simulink model "FinSimLagrange1"  (R2020b)
settings: Solver=FixedStepAuto  StartTime=0.0  StopTime=10.0  FixedStep=0.001  RelTol=1e-3
values from neighbouring files (symbols this model uses):
  m = {0 0 0 0 0}    [DynMatrixCalculator.m]    (also in DynMats_Iterative.mat = ; FinLagrange_2.m = mass{i})
  N = {zeros(3,1) zeros(3,1) zeros(3,1) zeros(3,1) zeros(3,1)}    [DynMatrixCalculator.m]    (also in DynMats_Iterative.mat = )
undefined symbols (not defined in the file or in its folder): X, Y, Z
libraries: sm_lib x34, nesl_utility x24
(part 3 of 4)

== matlab function FinSimLagrange1/Tau Iterative/MATLAB Function1 ==
  data: d2dt input; th2 input; th2dt input; th2ddt input; Force1 output; th3 input; th3dt input; th3ddt input; tau2 output; th4 input; th4dt input; th4ddt input; tau3 output; tau4 output
function [Force1, tau2, tau3, tau4] = fcn(d2dt, th2, th2dt, th2ddt, th3, th3dt, th3ddt, th4, th4dt, th4ddt)
% m0=cte(1); m1=cte(2); m2=cte(3); m3=cte(4); m4=cte(5); g=cte(6);
m0=40.117; m1=22.064; m2=9.805; m3=13.302; m4=10.723;
g=9.81;

%[Ixx Iyy Izz;Iyz Ixz Ixy]
Ic1=[13.366 13.428 .066;0 0 0];
Ic2=[.134 .165 .186;0 .001 -.012];
Ic3=[.082 .053 .058;-.001 0 0];
Ic4=[.048 .175 .153;0 .001 .003];
Ic5=[.018 .166 .164;0 -.001 .009];

Ixx0=Ic1(1,1);Ixx1=Ic2(1,1);Ixx2=Ic3(1,1);Ixx3=Ic4(1,1);Ixx4=Ic5(1,1);
Iyy0=Ic1(1,2);Iyy1=Ic2(1,2);Iyy2=Ic3(1,2);Iyy3=Ic4(1,2);Iyy4=Ic5(1,2);
Izz0=Ic1(1,3);Izz1=Ic2(1,3);Izz2=Ic3(1,3);Izz3=Ic4(1,3);Izz4=Ic5(1,3);
Iyz0=Ic1(2,1);Iyz1=Ic2(2,1);Iyz2=Ic3(2,1);Iyz3=Ic4(2,1);Iyz4=Ic5(2,1);
Ixz0=Ic1(2,2);Ixz1=Ic2(2,2);Ixz2=Ic3(2,2);Ixz3=Ic4(2,2);Ixz4=Ic5(2,2);
Ixy0=Ic1(2,3);Ixy1=Ic2(2,3);Ixy2=Ic3(2,3);Ixy3=Ic4(2,3);Ixy4=Ic5(2,3);

M=[0,                                                                                                                                                                                                                                                                                                                                                                                                                                                                                                                                                                      sin(th2)*(m3/1000 - m2/1000 + m4/1000) + cos(th2)*(m2/200 - (29*m3)/100 - (29*m4)/100 - (143*m4*cos(th3 + th4))/1000 + (3*m4*sin(th3 + th4))/200 + (11*m3*cos(th3))/1000 + (m4*cos(th3))/50 + (59*m3*sin(th3))/500 + (1913*m4*sin(th3))/5000),                                                                                                                                           (sin(th2)*(75*m4*cos(th3 + th4) + 715*m4*sin(th3 + th4) + 590*m3*cos(th3) + 1913*m4*cos(th3) - 55*m3*sin(th3) - 100*m4*sin(th3)))/5000,                                                                                                      (20674^(1/2)*m4*sin(th3 + th4 + atan(15/143))*sin(th2))/1000
0, Ixx3/2 + Ixx4/2 + Iyy3/2 + Iyy4/2 + Izz2 + (13*m2)/500000 + (17131*m3)/2500000 + (656439*m4)/10000000 - (13803*m3*cos(2*th3))/2000000 - (55477*m4*cos(2*th3))/1000000 - (Ixx4*cos(2*th3 + 2*th4))/2 + (Iyy4*cos(2*th3 + 2*th4))/2 + (649*m3*sin(2*th3))/500000 + (29*m4*sin(2*th3))/10000 + Ixy4*sin(2*th3 + 2*th4) + (158*m4*cos(2*th3 + 2*th4))/15625 - (429*m4*sin(2*th3 + 2*th4))/200000 + (4138563*m4*cos(th3 + th4))/100000000 - (86823*m4*sin(th3 + th4))/20000000 - (318351*m3*cos(th3))/100000000 + (59*m4*cos(th3))/5000000 + (7229*m4*cos(th4))/2000000 - (1707519*m3*sin(th3))/50000000 - (41937133*m4*sin(th3))/500000000 + (482409*m4*sin(th4))/10000000 - (12949*m4*cos(2*th3 + th4))/2000000 + (Ixx3*cos(2*th3))/2 - (Iyy3*cos(2*th3))/2 - (479409*m4*sin(2*th3 + th4))/10000000 - Ixy3*sin(2*th3), cos(th3)*(Ixz3 + (59*m3)/500000 + (1913*m4)/5000000 + Iyz4*cos(th4) + Ixz4*sin(th4) + (3*m4*cos(th4))/200000 + (143*m4*sin(th4))/1000000) - (sin(th3)*(1000000*Iyz3 + 11*m3 + 20*m4 - 1000000*Ixz4*cos(th4) + 1000000*Iyz4*sin(th4) - 143*m4*cos(th4) + 15*m4*sin(th4)))/1000000, sin(th3)*(cos(th4)*(Ixz4 + (143*m4)/1000000) - sin(th4)*(Iyz4 + (3*m4)/200000)) + cos(th3)*(cos(th4)*(Iyz4 + (3*m4)/200000) + sin(th4)*(Ixz4 + (143*m4)/1000000))
0,                                                                                                                                                                                                                                                                                                                                                                                                                                                                                                                                                                                          Iyz4*cos(th3 + th4) + Ixz4*sin(th3 + th4) + (3*m4*cos(th3 + th4))/200000 + Ixz3*cos(th3) + (143*m4*sin(th3 + th4))/1000000 - Iyz3*sin(th3) + (59*m3*cos(th3))/500000 + (29*m4*cos(th3))/100000 - (11*m3*sin(th3))/1000000,                                                                                                                                                                   Izz3 + Izz4 + (2809*m3)/200000 + (32907*m4)/250000 + (7229*m4*cos(th4))/1000000 + (482409*m4*sin(th4))/5000000,                                                                                     Izz4 + (10337*m4)/500000 + (87*m4*cos(th4))/20000 + (4147*m4*sin(th4))/100000
0,                                                                                                                                                                                                                                                                                                                                                                                                                                                                                                                                                                                                                                                                                                         Iyz4*cos(th3 + th4) + Ixz4*sin(th3 + th4) + (3*m4*cos(th3 + th4))/200000 + (143*m4*sin(th3 + th4))/1000000,                                                                                                                                                                                             Izz4 + (10337*m4)/500000 + (2879*m4*cos(th4))/1000000 + (275059*m4*sin(th4))/5000000,                                                                                                                                          Izz4 + (10337*m4)/500000];

V=[                                                                                                                                                                                                                                                                                  (m3*th2dt^2*cos(th2))/1000 - (m2*th2dt^2*cos(th2))/1000 + (m4*th2dt^2*cos(th2))/1000 - (m2*th2dt^2*sin(th2))/200 + (29*m3*th2dt^2*sin(th2))/100 + (29*m4*th2dt^2*sin(th2))/100 - (11*m3*th2dt^2*cos(th3)*sin(th2))/1000 - (11*m3*th3dt^2*cos(th3)*sin(th2))/1000 - (m4*th2dt^2*cos(th3)*sin(th2))/50 - (m4*th3dt^2*cos(th3)*sin(th2))/50 - (59*m3*th2dt^2*sin(th2)*sin(th3))/500 - (59*m3*th3dt^2*sin(th2)*sin(th3))/500 - (1913*m4*th2dt^2*sin(th2)*sin(th3))/5000 - (1913*m4*th3dt^2*sin(th2)*sin(th3))/5000 + (143*m4*th2dt^2*cos(th3)*cos(th4)*sin(th2))/1000 + (143*m4*th3dt^2*cos(th3)*cos(th4)*sin(th2))/1000 + (143*m4*th4dt^2*cos(th3)*cos(th4)*sin(th2))/1000 - (3*m4*th2dt^2*cos(th3)*sin(th2)*sin(th4))/200 - (3*m4*th2dt^2*cos(th4)*sin(th2)*sin(th3))/200 - (3*m4*th3dt^2*cos(th3)*sin(th2)*sin(th4))/200 - (3*m4*th3dt^2*cos(th4)*sin(th2)*sin(th3))/200 - (3*m4*th4dt^2*cos(th3)*sin(th2)*sin(th4))/200 - (3*m4*th4dt^2*cos(th4)*sin(th2)*sin(th3))/200 - (143*m4*th2dt^2*sin(th2)*sin(th3)*sin(th4))/1000 - (143*m4*th3dt^2*sin(th2)*sin(th3)*sin(th4))/1000 - (143*m4*th4dt^2*sin(th2)*sin(th3)*sin(th4))/1000 + (59*m3*th2dt*th3dt*cos(th2)*cos(th3))/250 + (1913*m4*th2dt*th3dt*cos(th2)*cos(th3))/2500 - (11*m3*th2dt*th3dt*cos(th2)*sin(th3))/500 - (m4*th2dt*th3dt*cos(th2)*sin(th3))/25 + (3*m4*th2dt*th3dt*cos(th2)*cos(th3)*cos(th4))/100 + (3*m4*th2dt*th4dt*cos(th2)*cos(th3)*cos(th4))/100 + (143*m4*th2dt*th3dt*cos(th2)*cos(th3)*sin(th4))/500 + (143*m4*th2dt*th3dt*cos(th2)*cos(th4)*sin(th3))/500 + (143*m4*th2dt*th4dt*cos(th2)*cos(th3)*sin(th4))/500 + (143*m4*th2dt*th4dt*cos(th2)*cos(th4)*sin(th3))/500 + (143*m4*th3dt*th4dt*cos(th3)*cos(th4)*sin(th2))/500 - (3*m4*th2dt*th3dt*cos(th2)*sin(th3)*sin(th4))/100 - (3*m4*th2dt*th4dt*cos(th2)*sin(th3)*sin(th4))/100 - (3*m4*th3dt*th4dt*cos(th3)*sin(th2)*sin(th4))/100 - (3*m4*th3dt*th4dt*cos(th4)*sin(th2)*sin(th3))/100 - (143*m4*th3dt*th4dt*sin(th2)*sin(th3)*sin(th4))/500
(29059*m3*th2dt^2)/100000000 + (29059*m4*th2dt^2)/100000000 + Ixz4*th3dt^2*cos(th3 + th4) + Ixz4*th4dt^2*cos(th3 + th4) - Iyz4*th3dt^2*sin(th3 + th4) - Iyz4*th4dt^2*sin(th3 + th4) + (143*m4*th3dt^2*cos(th3 + th4))/1000000 + (143*m4*th4dt^2*cos(th3 + th4))/1000000 - Iyz3*th3dt^2*cos(th3) - (3*m4*th3dt^2*sin(th3 + th4))/200000 - (3*m4*th4dt^2*sin(th3 + th4))/200000 - Ixz3*th3dt^2*sin(th3) - (11*m3*th3dt^2*cos(th3))/1000000 - (m4*th2dt^2*cos(th3))/50000 - (m4*th3dt^2*cos(th3))/50000 - (59*m3*th3dt^2*sin(th3))/500000 - (463*m4*th2dt^2*sin(th3))/5000000 - (1913*m4*th3dt^2*sin(th3))/5000000 - (29*m4*th2dt*th3dt)/5000 + Ixx4*th2dt*th3dt*sin(2*th3 + 2*th4) + Ixx4*th2dt*th4dt*sin(2*th3 + 2*th4) - Iyy4*th2dt*th3dt*sin(2*th3 + 2*th4) - Iyy4*th2dt*th4dt*sin(2*th3 + 2*th4) - (429*m4*th2dt*th3dt*cos(2*th3 + 2*th4))/100000 - (429*m4*th2dt*th4dt*cos(2*th3 + 2*th4))/100000 - (316*m4*th2dt*th3dt*sin(2*th3 + 2*th4))/15625 - (316*m4*th2dt*th4dt*sin(2*th3 + 2*th4))/15625 + 2*Ixz4*th3dt*th4dt*cos(th3 + th4) - 2*Iyz4*th3dt*th4dt*sin(th3 + th4) + (177*m4*th2dt*th3dt*cos(th3 + th4))/10000000 + (177*m4*th2dt*th4dt*cos(th3 + th4))/10000000 + (143*m4*th3dt*th4dt*cos(th3 + th4))/500000 + (8437*m4*th2dt*th3dt*sin(th3 + th4))/50000000 + (8437*m4*th2dt*th4dt*sin(th3 + th4))/50000000 - (3*m4*th3dt*th4dt*sin(th3 + th4))/100000 + (3481*m3*th2dt*th3dt*cos(th3))/25000000 + (112867*m4*th2dt*th3dt*cos(th3))/250000000 - (67709*m4*th2dt*th3dt*cos(th4))/5000000 + (4147*m4*th2dt*th4dt*cos(th4))/100000 - (649*m3*th2dt*th3dt*sin(th3))/50000000 - (59*m4*th2dt*th3dt*sin(th3))/2500000 - (1471*m4*th2dt*th3dt*sin(th4))/1000000 - (87*m4*th2dt*th4dt*sin(th4))/20000 - (479409*m4*th2dt*th3dt*cos(2*th3 + th4))/5000000 - (4147*m4*th2dt*th4dt*cos(2*th3 + th4))/100000 - 2*Ixy3*th2dt*th3dt*cos(2*th3) + (12949*m4*th2dt*th3dt*sin(2*th3 + th4))/1000000 + (87*m4*th2dt*th4dt*sin(2*th3 + th4))/20000 - Ixx3*th2dt*th3dt*sin(2*th3) + Iyy3*th2dt*th3dt*sin(2*th3) + (649*m3*th2dt*th3dt*cos(2*th3))/250000 + (29*m4*th2dt*th3dt*cos(2*th3))/5000 + 2*Ixy4*th2dt*th3dt*cos(2*th3 + 2*th4) + 2*Ixy4*th2dt*th4dt*cos(2*th3 + 2*th4) + (13803*m3*th2dt*th3dt*sin(2*th3))/1000000 + (55477*m4*th2dt*th3dt*sin(2*th3))/500000
                                                                                                                                                                                                                                                                                                                                                                                                                                                                                                                                                                                                                                                                                                                                                                                                                                                                                                                                                                                                                                                                                                                                                             (429*m4*th2dt^2*cos(2*th3 + 2*th4))/200000 - (29*m4*th3dt^2)/5000 - (29*m4*th2dt^2)/10000 + (158*m4*th2dt^2*sin(2*th3 + 2*th4))/15625 + (87*m4*th2dt^2*cos(th3 + th4))/20000 + (4147*m4*th2dt^2*sin(th3 + th4))/100000 + (1711*m3*th2dt^2*cos(th3))/50000 + (841*m4*th2dt^2*cos(th3))/10000 - (67709*m4*th2dt^2*cos(th4))/10000000 - (67709*m4*th3dt^2*cos(th4))/5000000 + (4147*m4*th4dt^2*cos(th4))/100000 - (319*m3*th2dt^2*sin(th3))/100000 - (1471*m4*th2dt^2*sin(th4))/2000000 - (1471*m4*th3dt^2*sin(th4))/1000000 - (87*m4*th4dt^2*sin(th4))/20000 + (479409*m4*th2dt^2*cos(2*th3 + th4))/10000000 + Ixy3*th2dt^2*cos(2*th3) - (12949*m4*th2dt^2*sin(2*th3 + th4))/2000000 + (Ixx3*th2dt^2*sin(2*th3))/2 - (Iyy3*th2dt^2*sin(2*th3))/2 - (649*m3*th2dt^2*cos(2*th3))/500000 - (29*m4*th2dt^2*cos(2*th3))/10000 - Ixy4*th2dt^2*cos(2*th3 + 2*th4) - (13803*m3*th2dt^2*sin(2*th3))/2000000 - (55477*m4*th2dt^2*sin(2*th3))/1000000 - (Ixx4*th2dt^2*sin(2*th3 + 2*th4))/2 + (Iyy4*th2dt^2*sin(2*th3 + 2*th4))/2 + (4147*m4*th3dt*th4dt*cos(th4))/50000 - (87*m4*th3dt*th4dt*sin(th4))/10000
                                                                                                                                                                                                                                                                                                                                                                                                                                                                                                                                                                                                                                                                                                                                                                                                                                                                                                                                                                                                                                                                                                                                                                                                                                                                                                                                                                                                                                                                                                                                                                                                                                                                                                                  (429*m4*th2dt^2*cos(2*th3 + 2*th4))/200000 + (158*m4*th2dt^2*sin(2*th3 + 2*th4))/15625 + (87*m4*th2dt^2*cos(th3 + th4))/20000 + (4147*m4*th2dt^2*sin(th3 + th4))/100000 - (275059*m4*th2dt^2*cos(th4))/10000000 - (275059*m4*th3dt^2*cos(th4))/5000000 + (2879*m4*th2dt^2*sin(th4))/2000000 + (2879*m4*th3dt^2*sin(th4))/1000000 + (272059*m4*th2dt^2*cos(2*th3 + th4))/10000000 - (8599*m4*th2dt^2*sin(2*th3 + th4))/2000000 - Ixy4*th2dt^2*cos(2*th3 + 2*th4) - (Ixx4*th2dt^2*sin(2*th3 + 2*th4))/2 + (Iyy4*th2dt^2*sin(2*th3 + 2*th4))/2];

G=[                                                                                                            0
                                                                                                            0
-(g*(15*m4*sin(th3 + th4) - 143*m4*cos(th3 + th4) + 11*m3*cos(th3) + 118*m3*sin(th3) + 290*m4*sin(th3)))/1000
                                                         (g*m4*(143*cos(th3 + th4) - 15*sin(th3 + th4)))/1000];

Force1=cos(th2)*(m4*((th2dt*cos(th3)*cos(th4) - th2dt*sin(th3)*sin(th4))*((3*th3dt)/200 + (3*th4dt)/200 + (th2dt*cos(th3)*cos(th4))/1000 - (th2dt*sin(th3)*sin(th4))/1000) - (29*th2ddt)/100 + (th2dt*cos(th3)*sin(th4) + th2dt*cos(th4)*sin(th3))*((143*th3dt)/1000 + (143*th4dt)/1000 + (th2dt*cos(th3)*sin(th4))/1000 + (th2dt*cos(th4)*sin(th3))/1000) + (143*th4dt*(th2dt*cos(th3)*sin(th4) + th2dt*cos(th4)*sin(th3)))/1000 + (3*th4dt*(th2dt*cos(th3)*cos(th4) - th2dt*sin(th3)*sin(th4)))/200 + (3*cos(th4)*(th2ddt*sin(th3) + th2dt*th3dt*cos(th3)))/200 - (143*cos(th4)*(th2ddt*cos(th3) - th2dt*th3dt*sin(th3)))/1000 + (143*sin(th4)*(th2ddt*sin(th3) + th2dt*th3dt*cos(th3)))/1000 + (3*sin(th4)*(th2ddt*cos(th3) - th2dt*th3dt*sin(th3)))/200 + d2dt*cos(th2) + (th2ddt*cos(th3))/50 + (1913*th2ddt*sin(th3))/5000 + (1913*th2dt*th3dt*cos(th3))/2500 - (th2dt*th3dt*sin(th3))/25) + m3*(d2dt*cos(th2) - (29*th2ddt)/100 + (11*th2ddt*cos(th3))/1000 + (59*th2ddt*sin(th3))/500 + (59*th2dt*th3dt*cos(th3))/500 - (11*th2dt*th3dt*sin(th3))/1000 + th2dt*cos(th3)*((59*th3dt)/500 + (th2dt*cos(th3))/1000) - th2dt*sin(th3)*((11*th3dt)/1000 - (th2dt*sin(th3))/1000)) + m2*(- th2dt^2/1000 + th2ddt/200 + d2dt*cos(th2))) + d2dt*m1 + sin(th2)*(cos(th3)*(m4*cos(th4)*((3*th3ddt)/200 + (3*th4ddt)/200 - cos(th4)*(th3dt^2/50 - (1913*th3ddt)/5000 - cos(th3)*((29*th2dt^2)/100 + d2dt*sin(th2)) + g*sin(th3) + th2dt*cos(th3)*((th2dt*cos(th3))/50 + (1913*th2dt*sin(th3))/5000)) + sin(th4)*((1913*th3dt^2)/5000 + th3ddt/50 - sin(th3)*((29*th2dt^2)/100 + d2dt*sin(th2)) - g*cos(th3) + th2dt*sin(th3)*((th2dt*cos(th3))/50 + (1913*th2dt*sin(th3))/5000)) - (th4dt*(th2dt*cos(th3)*sin(th4) + th2dt*cos(th4)*sin(th3)))/1000 + (cos(th4)*(th2ddt*cos(th3) - th2dt*th3dt*sin(th3)))/1000 - (sin(th4)*(th2ddt*sin(th3) + th2dt*th3dt*cos(th3)))/1000 - (th2dt*cos(th3)*cos(th4) - th2dt*sin(th3)*sin(th4))*((3*th2dt*cos(th3)*sin(th4))/200 - (143*th2dt*cos(th3)*cos(th4))/1000 + (3*th2dt*cos(th4)*sin(th3))/200 + (143*th2dt*sin(th3)*sin(th4))/1000) + (th3dt + th4dt)*((143*th3dt)/1000 + (143*th4dt)/1000 + (th2dt*cos(th3)*sin(th4))/1000 + (th2dt*cos(th4)*sin(th3))/1000)) - m3*(g*sin(th3) - cos(th3)*((29*th2dt^2)/100 + d2dt*sin(th2)) - (th2ddt*cos(th3))/1000 - (59*th3ddt)/500 + th3dt*((11*th3dt)/1000 - (th2dt*sin(th3))/1000) + (th2dt*th3dt*sin(th3))/1000 + th2dt*cos(th3)*((11*th2dt*cos(th3))/1000 + (59*th2dt*sin(th3))/500)) + m4*sin(th4)*((143*th3ddt)/1000 + (143*th4ddt)/1000 - sin(th4)*(th3dt^2/50 - (1913*th3ddt)/5000 - cos(th3)*((29*th2dt^2)/100 + d2dt*sin(th2)) + g*sin(th3) + th2dt*cos(th3)*((th2dt*cos(th3))/50 + (1913*th2dt*sin(th3))/5000)) - cos(th4)*((1913*th3dt^2)/5000 + th3ddt/50 - sin(th3)*((29*th2dt^2)/100 + d2dt*sin(th2)) - g*cos(th3) + th2dt*sin(th3)*((th2dt*cos(th3))/50 + (1913*th2dt*sin(th3))/5000)) + (th4dt*(th2dt*cos(th3)*cos(th4) - th2dt*sin(th3)*sin(th4)))/1000 + (cos(th4)*(th2ddt*sin(th3) + th2dt*th3dt*cos(th3)))/1000 + (sin(th4)*(th2ddt*cos(th3) - th2dt*th3dt*sin(th3)))/1000 - (th2dt*cos(th3)*sin(th4) + th2dt*cos(th4)*sin(th3))*((3*th2dt*cos(th3)*sin(th4))/200 - (143*th2dt*cos(th3)*cos(th4))/1000 + (3*th2dt*cos(th4)*sin(th3))/200 + (143*th2dt*sin(th3)*sin(th4))/1000) - (th3dt + th4dt)*((3*th3dt)/200 + (3*th4dt)/200 + (th2dt*cos(th3)*cos(th4))/1000 - (th2dt*sin(th3)*sin(th4))/1000))) + sin(th3)*(m3*(sin(th3)*((29*th2dt^2)/100 + d2dt*sin(th2)) - (11*th3ddt)/1000 + g*cos(th3) - th3dt*((59*th3dt)/500 + (th2dt*cos(th3))/1000) + (th2ddt*sin(th3))/1000 + (th2dt*th3dt*cos(th3))/1000 - th2dt*sin(th3)*((11*th2dt*cos(th3))/1000 + (59*th2dt*sin(th3))/500)) + m4*cos(th4)*((143*th3ddt)/1000 + (143*th4ddt)/1000 - sin(th4)*(th3dt^2/50 - (1913*th3ddt)/5000 - cos(th3)*((29*th2dt^2)/100 + d2dt*sin(th2)) + g*sin(th3) + th2dt*cos(th3)*((th2dt*cos(th3))/50 + (1913*th2dt*sin(th3))/5000)) - cos(th4)*((1913*th3dt^2)/5000 + th3ddt/50 - sin(th3)*((29*th2dt^2)/100 + d2dt*sin(th2)) - g*cos(th3) + th2dt*sin(th3)*((th2dt*cos(th3))/50 + (1913*th2dt*sin(th3))/5000)) + (th4dt*(th2dt*cos(th3)*cos(th4) - th2dt*sin(th3)*sin(th4)))/1000 + (cos(th4)*(th2ddt*sin(th3) + th2dt*th3dt*cos(th3)))/1000 + (sin(th4)*(th2ddt*cos(th3) - th2dt*th3dt*sin(th3)))/1000 - (th2dt*cos(th3)*sin(th4) + th2dt*cos(th4)*sin(th3))*((3*th2dt*cos(th3)*sin(th4))/200 - (143*th2dt*cos(th3)*cos(th4))/1000 + (3*th2dt*cos(th4)*sin(th3))/200 + (143*th2dt*sin(th3)*sin(th4))/1000) - (th3dt + th4dt)*((3*th3dt)/200 + (3*th4dt)/200 + (th2dt*cos(th3)*cos(th4))/1000 - (th2dt*sin(th3)*sin(th4))/1000)) - m4*sin(th4)*((3*th3ddt)/200 + (3*th4ddt)/200 - cos(th4)*(th3dt^2/50 - (1913*th3ddt)/5000 - cos(th3)*((29*th2dt^2)/100 + d2dt*sin(th2)) + g*sin(th3) + th2dt*cos(th3)*((th2dt*cos(th3))/50 + (1913*th2dt*sin(th3))/5000)) + sin(th4)*((1913*th3dt^2)/5000 + th3ddt/50 - sin(th3)*((29*th2dt^2)/100 + d2dt*sin(th2)) - g*cos(th3) + th2dt*sin(th3)*((th2dt*cos(th3))/50 + (1913*th2dt*sin(th3))/5000)) - (th4dt*(th2dt*cos(th3)*sin(th4) + th2dt*cos(th4)*sin(th3)))/1000 + (cos(th4)*(th2ddt*cos(th3) - th2dt*th3dt*sin(th3)))/1000 - (sin(th4)*(th2ddt*sin(th3) + th2dt*th3dt*cos(th3)))/1000 - (th2dt*cos(th3)*cos(th4) - th2dt*sin(th3)*sin(th4))*((3*th2dt*cos(th3)*sin(th4))/200 - (143*th2dt*cos(th3)*cos(th4))/1000 + (3*th2dt*cos(th4)*sin(th3))/200 + (143*th2dt*sin(th3)*sin(th4))/1000) + (th3dt + th4dt)*((143*th3dt)/1000 + (143*th4dt)/1000 + (th2dt*cos(th3)*sin(th4))/1000 + (th2dt*cos(th4)*sin(th3))/1000))) - m2*(th2dt^2/200 + th2ddt/1000 - d2dt*sin(th2)));

x=(1913*cos(th2)*cos(th3)*cos(th4))/5000 - (29*cos(th2)*sin(th3))/100 - (1913*cos(th2)*sin(th3)*sin(th4))/5000 - (59*cos(th2))/100000 - (cos(th2)*cos(th3)*sin(th4))/50 - (cos(th2)*cos(th4)*sin(th3))/50;
y=(29*cos(th3))/100 + (cos(th3)*cos(th4))/50 + (1913*cos(th3)*sin(th4))/5000 + (1913*cos(th4)*sin(th3))/5000 - (sin(th3)*sin(th4))/50 + 873/2500;
z=(59*sin(th2))/100000 + (29*sin(th2)*sin(th3))/100 + (cos(th3)*sin(th2)*sin(th4))/50 + (cos(th4)*sin(th2)*sin(th3))/50 + (1913*sin(th2)*sin(th3)*sin(th4))/5000 - (1913*cos(th3)*cos(th4)*sin(th2))/5000;

th1ddt=0;
T=M*[th1ddt;th2ddt;th3ddt;th4ddt]+V+G;
tau2=T(2); tau3=T(3); tau4=T(4);
